simulink model "SF101A_MotQuadDetn"  (R2013b)
settings: Solver=FixedStepDiscrete  StartTime=0.0  StopTime=1  FixedStep=Ts  RelTol=1e-3
model workspace (MAT data in the model file):
  SLAMConfig_1_ATPP = [3707764736; 2; 1; 1; 1; 34]
values from neighbouring files (symbols this model uses):
  MotQuadDetnMotDirHysInsts = DataDict.Calibration    [SF101A_MotQuadDetn_DataDict.m]
  MOTTQCMDTOLR_MOTNWTMTR_F32 = DataDict.Constant    [SF101A_MotQuadDetn_DataDict.m]
undefined symbols (not defined in the file or in its folder): MotQuad1
libraries: simulink x5, NxtrAbslt x2, NxtrSign x2
(part 2 of 2)

== system SF101A_MotQuadDetn/MotQuadDetn/MotQuadDetnPer1/Determine_Motor_Quadrant/Quads 2//4 Change in direction/If Action Subsystem1 ==
  In1 : Inport
  Action Port : ActionPort  ActionType=else
  CopyRight2 : Subsystem  Description=|  mask(Copyright Information){none=on}
      | Copyright info block.                                               
      |                                                                     
      | Place copyright information at the top of every subsystem in design.
      mask prompts: none "No parameters"
      mask help: Place copyright information at the top of every subsystem in design.
      mask Display:
      | NxtrConf = 'Nexteer Confidential';
      | 
      | sys = bdroot; %handle for the current model ("system")
      | first = get_param(sys,'Created');
      | if(isempty(first))
      |     first = datestr(now,'yyyy');
      | else
      |     first = first(end-3:end);  %year is last four digits
      | end
      | 
      | last = get_param(sys,'LastModifiedDate');
      | if isempty(last)
      |     last = datestr(now,'yyyy');
      | else
      |     last = last(end-3:end);
      | end
      | 
      | if strcmp(first,last)
      |     fprintf('%s -- Copyright %s Nexteer',NxtrConf,first)
      | else
      |     fprintf('%s -- %s%s- %s Nexteer',NxtrConf,char(169),first,last)
      | end
  Out1 : Outport
  wires:
  In1/1 -> Out1/1

== system SF101A_MotQuadDetn/MotQuadDetn/MotQuadDetnPer1/Determine_TqCmd_Sign/Determine Motor Torque Command Sign/CopyRight2 ==

== system SF101A_MotQuadDetn/MotQuadDetn/MotQuadDetnPer1/Determine_TqCmd_Sign/Determine Motor Torque Command Sign1/CopyRight2 ==

== system SF101A_MotQuadDetn/MotQuadDetn/MotQuadDetnPer1/Determine_Motor_Quadrant/Quads 1//3 No change in direction/If Action Subsystem/CopyRight2 ==

== system SF101A_MotQuadDetn/MotQuadDetn/MotQuadDetnPer1/Determine_Motor_Quadrant/Quads 1//3 No change in direction/If Action Subsystem1/CopyRight2 ==

== system SF101A_MotQuadDetn/MotQuadDetn/MotQuadDetnPer1/Determine_Motor_Quadrant/Quads 2//4 Change in direction/If Action Subsystem/CopyRight2 ==

== system SF101A_MotQuadDetn/MotQuadDetn/MotQuadDetnPer1/Determine_Motor_Quadrant/Quads 2//4 Change in direction/If Action Subsystem1/CopyRight2 ==
